simulink model "q_aero_2dof_lqr_control"  (R2017a)
settings: Solver=ode1  StartTime=0.0  StopTime=inf  FixedStep=0.002  RelTol=1e-3  EnableMultiTasking=on
PreLoadFcn:
  | quanser_aero_lqr
libraries: simulink_extras x4, quarc_library x3, quanser_aero x1
settings Model: SimulationMode=external  ExtModeTrigDuration=15000  Creator=MLevis  LastModifiedBy=Administrator
settings SolverCC: PositivePriorityOrder=on
settings DataIOCC: LimitDataPoints=on  SaveFormat=Array
settings OptimizationCC: LifeSpan=inf
settings DebuggingCC: SolverPrmCheckMsg=warning  SFUnexpectedBacktrackingDiag=warning  SFNoUnconditionalDefaultTransitionDiag=warning  SFExecutionAtInitializationDiag=none
settings HardwareCC: ProdBitPerPointer=32  ProdBitPerSizeT=32  ProdBitPerPtrDiffT=32  ProdLargestAtomicFloat=None  ProdIntDivRoundTo=Undefined  ProdEndianess=Unspecified  ProdWordSize=32  ProdHWDeviceType=32-bit Generic
settings ModelReferenceCC: PropagateSignalLabelsOutOfModel=off
settings RTWCC: SystemTargetFile=quarc_win64.tlc  TemplateMakefile=quarc_default_tmf  Description=QUARC Win64 Target
settings STFCustomTargetCC: TargetPreCompLibLocation=C:\PROGRA~3\QUARC\lib\2014a\win64\release  ConcurrentExecutionCompliant=on  GeneratePreprocessorConditionals=Disable all  SystemTargetFile=quarc_win64.tlc
settings GRTTargetCC: TargetPreCompLibLocation=C:\PROGRA~3\QUARC\lib\2014a\win64\release  TargetLangStandard=C89/C90 (ANSI)  ParMdlRefBuildCompliant=off  CompOptLevelCompliant=off  GeneratePreprocessorConditionals=Disable all  CombineOutputUpdateFcns=off  MatFileLogging=off  CPPClassGenCompliant=off  GRTInterface=on  UseToolchainInfoCompliant=off  ExtMode=on  ExtModeMexFile=quarc_comm
settings ConfigComp: CovMetricSettings=dw  CovHtmlReporting=on  CovSaveCumulativeToWorkspaceVar=on  CovSaveSingleToWorkspaceVar=on  CovExternalEMLEnable=off  CovSFcnEnable=off

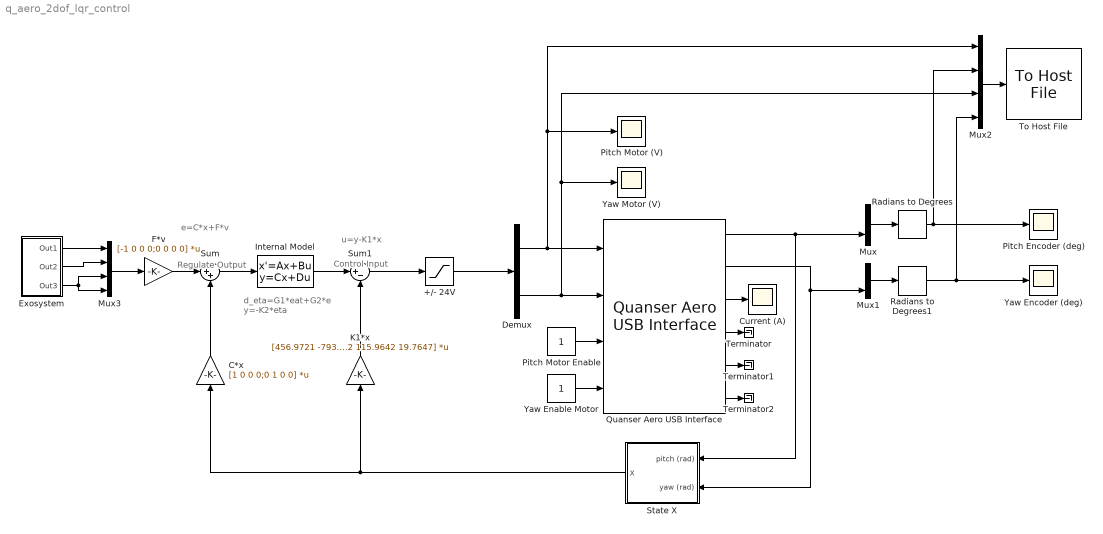
== system q_aero_2dof_lqr_control ==
  note: u=y-K1*x
  note: Control Input
  note: e=C*x+F*v
  note: Regulate Output
  note: d_eta=G1*eat+G2*e
      |        y=-K2*eta
  +/- 24V : Saturate  UpperLimit=24  LowerLimit=-24
  C*x : Gain  Gain=[1 0 0 0;0 1 0 0]  Multiplication=Matrix(K*u)
  Current (A) : Scope
  Demux : Demux  Outputs=2
  Exosystem : Subsystem
  F*v : Gain  Gain=[-1 0 0 0;0 0 0 0]  Multiplication=Matrix(K*u)
  "Internal Model " : StateSpace  A=[0 1 0 0 0 0;0 0 1 0 0 0;0 -1 0 0 0 0;0 0 0 0 1 0;0 0 0 0 0 1;0 0 0 0 -1 0]  B=[0 0;0 0;1 0;0 0;0 0;0 1]  C=[-139.1 -1888 -1334.1 5664.7 5615 3110.8;-4892.1 -5540.6 -3198.1 2116.5 577.4 57.8]  D=[0 0;0 0]  X0=[1 0 2 1 0 2]
  K1*x : Gain  Gain=[456.9721 -793.3427 70.3033 -98.0538;856.0024 97.9162 115.9642 19.7647]  Multiplication=Matrix(K*u)
  Mux : Mux  Inputs=2
  Mux1 : Mux  Inputs=2
  Mux2 : Mux
  Mux3 : Mux
  Pitch Encoder (deg) : Scope
  Pitch Motor (V) : Scope
  Pitch Motor Enable : Constant
  Quanser Aero USB Interface : quanser_aero/Quanser Aero USB Interface
  Radians to Degrees : simulink_extras/Transformations/Radians to Degrees
  Radians to Degrees1 : simulink_extras/Transformations/Radians to Degrees
  State X : Subsystem
  Sum : Sum  Inputs=|++
  Sum1 : Sum  Inputs=|+-
  Terminator : Terminator
  Terminator1 : Terminator
  Terminator2 : Terminator
  To Host File : quarc_library/Sinks/To Host/To Host File  file_name=aero_lqr_rsp.mat  variable_name=lqr_rsp  decimation=1  sample_time=-1  file_format=MAT-file v.4  options=No header or footer  append=off  final_file_name=aero_lqr_rsp.mat
  Yaw Enable Motor : Constant
  Yaw Encoder (deg) : Scope
  Yaw Motor (V) : Scope
  wires:
  Mux/1 -> Radians to Degrees/1
  Radians to Degrees/1 -> Mux2/2, Pitch Encoder (deg)/1
  Radians to Degrees1/1 -> Mux2/4, Yaw Encoder (deg)/1
  Pitch Motor Enable/1 -> Quanser Aero USB Interface/3
  Yaw Enable Motor/1 -> Quanser Aero USB Interface/4
  Demux/2 -> Quanser Aero USB Interface/2, Mux2/3, Yaw Motor (V)/1
  Mux1/1 -> Radians to Degrees1/1
  Mux3/1 -> F*v/1
  +/- 24V/1 -> Demux/1
  Quanser Aero USB Interface/3 -> Current (A)/1
  Quanser Aero USB Interface/1 -> Mux/2, State X/1(pitch (rad))
  Quanser Aero USB Interface/2 -> Mux1/2, State X/2(yaw (rad))
  Quanser Aero USB Interface/4 -> Terminator/1
  Quanser Aero USB Interface/5 -> Terminator1/1
  Quanser Aero USB Interface/6 -> Terminator2/1
  Mux2/1 -> To Host File/1
  Demux/1 -> Quanser Aero USB Interface/1, Mux2/1, Pitch Motor (V)/1
  Exosystem/1(Out1) -> Mux3/1
  Exosystem/3(Out3) -> Mux3/3, Mux3/4
  Exosystem/2(Out2) -> Mux3/2
  F*v/1 -> Sum/1
  State X/1(X) -> K1*x/1, C*x/1
  Sum/1 -> "Internal Model "/1
  C*x/1 -> Sum/2
  "Internal Model "/1 -> Sum1/1
  K1*x/1 -> Sum1/2
  Sum1/1 -> +/- 24V/1

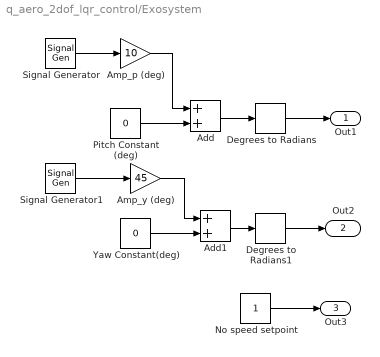
== system q_aero_2dof_lqr_control/Exosystem ==
  Add : Sum
  Add1 : Sum
  Amp_p (deg) : Gain  Gain=10
  Amp_y (deg) : Gain  Gain=45
  Degrees to Radians : simulink_extras/Transformations/Degrees to Radians
  Degrees to Radians1 : simulink_extras/Transformations/Degrees to Radians
  No speed setpoint : Constant
  Pitch Constant (deg) : Constant  Value=0
  Signal Generator : SignalGenerator  Frequency=0.1
  Signal Generator1 : SignalGenerator  Frequency=0.04
  Yaw Constant(deg) : Constant  Value=0
  Out1 : Outport
  Out2 : Outport  Port=2
  Out3 : Outport  Port=3
  wires:
  Signal Generator1/1 -> Amp_y (deg)/1
  Signal Generator/1 -> Amp_p (deg)/1
  Add/1 -> Degrees to Radians/1
  Yaw Constant(deg)/1 -> Add1/2
  Add1/1 -> Degrees to Radians1/1
  Pitch Constant (deg)/1 -> Add/2
  Degrees to Radians/1 -> Out1/1
  Amp_p (deg)/1 -> Add/1
  Amp_y (deg)/1 -> Add1/1
  No speed setpoint/1 -> Out3/1
  Degrees to Radians1/1 -> Out2/1

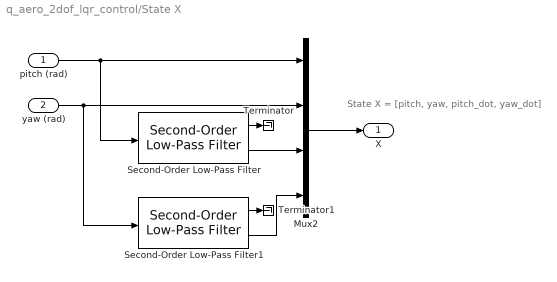
== system q_aero_2dof_lqr_control/State X ==
  note: State X = [pitch, yaw, pitch_dot, yaw_dot]
  pitch (rad) : Inport
  yaw (rad) : Inport  Port=2
  Mux2 : Mux
  Second-Order Low-Pass Filter : quarc_library/Continuous/Second-Order Low-Pass Filter  params_source=Internal (dialog parameters)  input_width=50  input_zeta=0.8  input_init=0
  Second-Order Low-Pass Filter1 : quarc_library/Continuous/Second-Order Low-Pass Filter  params_source=Internal (dialog parameters)  input_width=50  input_zeta=0.8  input_init=0
  Terminator : Terminator
  Terminator1 : Terminator
  X : Outport
  wires:
  Mux2/1 -> X/1
  yaw (rad)/1 -> Second-Order Low-Pass Filter1/1, Mux2/2
  pitch (rad)/1 -> Second-Order Low-Pass Filter/1, Mux2/1
  Second-Order Low-Pass Filter/2 -> Mux2/3
  Second-Order Low-Pass Filter1/2 -> Mux2/4
  Second-Order Low-Pass Filter/1 -> Terminator/1
  Second-Order Low-Pass Filter1/1 -> Terminator1/1
